simulink model "twip_control_KMLOGIC"  (R2018a)
settings: Solver=ode45  StartTime=0.0  StopTime=10  RelTol=1e-3  EnableMultiTasking=on
values from neighbouring files (symbols this model uses):
  MFM = MFM*length(Centers(i).C)    [Tilt_RuleBase.m]    (also in Yaw_RuleBase.m)
  RulesTILT = [NB NB NB NB NM NS ZR ... (first row only)    [Tilt_RuleBase.m]
  RulesYAW = [NB NB NB NB NM NS ZR ... (first row only)    [Yaw_RuleBase.m]
undefined symbols (not defined in the file or in its folder): CentersTILT, CentersYAW, KMLOGIC
libraries: simulink x2
settings Model: Creator=elew  LastModifiedBy=mattclark
settings DataIOCC: LimitDataPoints=on  SaveFormat=Array
settings OptimizationCC: BlockReduction=off  OptimizeBlockIOStorage=off  BufferReuse=off  GlobalBufferReuse=off  ExpressionFolding=off  LocalBlockOutputs=off  LifeSpan=inf  OptimizeDataStoreBuffers=off  BusAssignmentInplaceUpdate=off
settings DebuggingCC: SFUnexpectedBacktrackingDiag=warning  SFNoUnconditionalDefaultTransitionDiag=warning  SFExecutionAtInitializationDiag=none
settings HardwareCC: ProdBitPerPointer=32  ProdBitPerSizeT=32  ProdBitPerPtrDiffT=32  ProdLargestAtomicFloat=None  ProdIntDivRoundTo=Undefined  ProdEndianess=Unspecified  ProdWordSize=32  ProdHWDeviceType=32-bit Generic
settings ModelReferenceCC: PropagateSignalLabelsOutOfModel=off
settings CodeAppCC: StateflowObjectComments=on
settings GRTTargetCC: TargetLangStandard=C89/C90 (ANSI)  GeneratePreprocessorConditionals=Disable all
settings ConfigComp: CovMetricSettings=dw  CovHtmlReporting=on  CovSaveCumulativeToWorkspaceVar=on  CovSaveSingleToWorkspaceVar=on  CovExternalEMLEnable=off
settings ConfigurationSet: Description=SimMechanics 2G

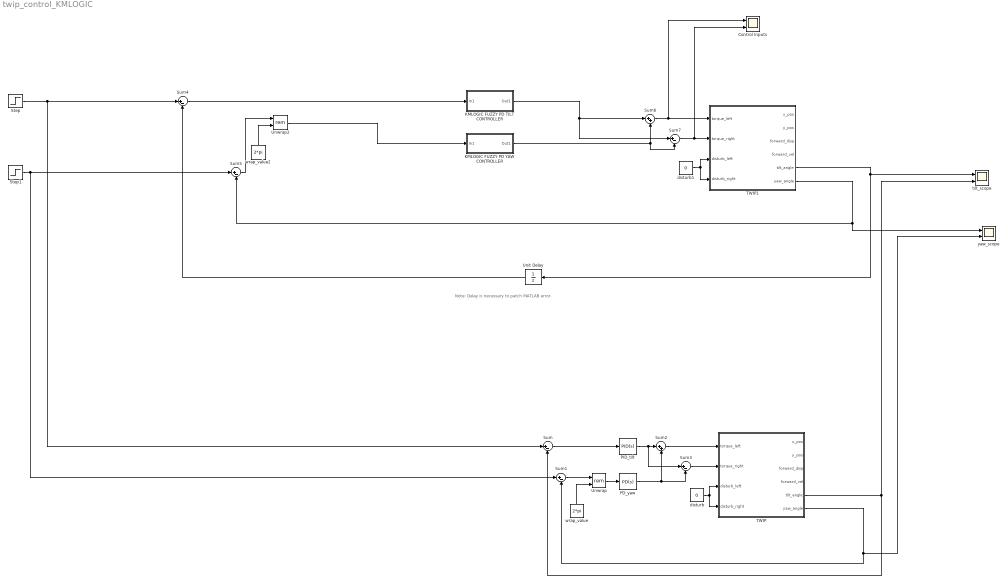
== system twip_control_KMLOGIC ==
  note: Note: Delay is necessary to patch MATLAB error.
  Control Inputs : Scope  NumInputPorts=2
  "KMLOGIC FUZZY PD TILT CONTROLLER " : Subsystem
  KMLOGIC FUZZY PD YAW CONTROLLER : Subsystem
  PD_yaw : simulink/Continuous/PID Controller  Controller=PD  TimeDomain=Continuous-time  SampleTime=-1  IntegratorMethod=Forward Euler  FilterMethod=Forward Euler  Form=Parallel  UseFilter=on  ControllerParametersSource=internal  P=25  I=100  D=1  N=100  InitialConditionSource=internal  InitialConditionForIntegrator=0  InitialConditionForFilter=0  ExternalReset=none  LimitOutput=off  UpperSaturationLimit=inf  LowerSaturationLimit=-inf  LinearizeAsGain=on  AntiWindupMode=none  Kb=1  TrackingMode=off  Kt=1  PParamMin=[]  PParamMax=[]  IParamMin=[]  IParamMax=[]  DParamMin=[]  DParamMax=[]  NParamMin=[]  NParamMax=[]  KbParamMin=[]  KbParamMax=[]  KtParamMin=[]  KtParamMax=[]  POutMin=[]  POutMax=[]  IOutMin=[]  IOutMax=[]  DOutMin=[]  DOutMax=[]  NOutMin=[]  NOutMax=[]  KbOutMin=[]  KbOutMax=[]  KtOutMin=[]  KtOutMax=[]  IntegratorOutMin=[]  IntegratorOutMax=[]  FilterOutMin=[]  FilterOutMax=[]  SumOutMin=[]  SumOutMax=[]  SumI1OutMin=[]  SumI1OutMax=[]  SumI2OutMin=[]  SumI2OutMax=[]  SumI3OutMin=[]  SumI3OutMax=[]  SumDOutMin=[]  SumDOutMax=[]  SaturationOutMin=[]  SaturationOutMax=[]  IntegratorContinuousStateAttributes=''  IntegratorStateMustResolveToSignalObject=off  IntegratorRTWStateStorageClass=Auto  FilterContinuousStateAttributes=''  FilterStateMustResolveToSignalObject=off  FilterRTWStateStorageClass=Auto  DifferentiatorICPrevScaledInput=0  DifferentiatorOutMin=[]  DifferentiatorOutMax=[]  FilterDiffOutCoefMin=[]  FilterDiffOutCoefMax=[]  SumDenOutMin=[]  SumDenOutMax=[]  SumNumOutMin=[]  SumNumOutMax=[]  ReciprocalOutMin=[]  ReciprocalOutMax=[]  DivideOutMin=[]  DivideOutMax=[]  TunerSelectOption=Transfer Function Based (PID Tuner App)
  PID_tilt : simulink/Continuous/PID Controller  Controller=PID  TimeDomain=Continuous-time  SampleTime=-1  IntegratorMethod=Forward Euler  FilterMethod=Forward Euler  Form=Parallel  UseFilter=on  ControllerParametersSource=internal  P=50  I=100  D=2  N=100  InitialConditionSource=internal  InitialConditionForIntegrator=0  InitialConditionForFilter=0  ExternalReset=none  LimitOutput=off  UpperSaturationLimit=inf  LowerSaturationLimit=-inf  LinearizeAsGain=on  AntiWindupMode=none  Kb=1  TrackingMode=off  Kt=1  PParamMin=[]  PParamMax=[]  IParamMin=[]  IParamMax=[]  DParamMin=[]  DParamMax=[]  NParamMin=[]  NParamMax=[]  KbParamMin=[]  KbParamMax=[]  KtParamMin=[]  KtParamMax=[]  POutMin=[]  POutMax=[]  IOutMin=[]  IOutMax=[]  DOutMin=[]  DOutMax=[]  NOutMin=[]  NOutMax=[]  KbOutMin=[]  KbOutMax=[]  KtOutMin=[]  KtOutMax=[]  IntegratorOutMin=[]  IntegratorOutMax=[]  FilterOutMin=[]  FilterOutMax=[]  SumOutMin=[]  SumOutMax=[]  SumI1OutMin=[]  SumI1OutMax=[]  SumI2OutMin=[]  SumI2OutMax=[]  SumI3OutMin=[]  SumI3OutMax=[]  SumDOutMin=[]  SumDOutMax=[]  SaturationOutMin=[]  SaturationOutMax=[]  IntegratorContinuousStateAttributes=''  IntegratorStateMustResolveToSignalObject=off  IntegratorRTWStateStorageClass=Auto  FilterContinuousStateAttributes=''  FilterStateMustResolveToSignalObject=off  FilterRTWStateStorageClass=Auto  DifferentiatorICPrevScaledInput=0  DifferentiatorOutMin=[]  DifferentiatorOutMax=[]  FilterDiffOutCoefMin=[]  FilterDiffOutCoefMax=[]  SumDenOutMin=[]  SumDenOutMax=[]  SumNumOutMin=[]  SumNumOutMax=[]  ReciprocalOutMin=[]  ReciprocalOutMax=[]  DivideOutMin=[]  DivideOutMax=[]  TunerSelectOption=Transfer Function Based (PID Tuner App)
  Step : Step  After=-0.3  SampleTime=0
  Step1 : Step  After=0.1  SampleTime=0
  Sum{,1,3..5,7} (6 alike) : Sum  Inputs=|+-
  Sum2 : Sum  Inputs=|++
  Sum6 : Sum  Inputs=|++
  TWIP : Subsystem
      mask Display:
      | image('twip_mask.png')
      | port_label('input', 1, 'torque_l')
      | port_label('input', 2, 'torque_r')
      | port_label('input', 3, 'disturb_l')
      | port_label('input', 4, 'disturb_r')
      | 
      | 
      | port_label('output', 1, 'x_pos')
      | port_label('output', 2, 'y_pos')
      | port_label('output', 3, 'disp')
      | port_label('output', 4, 'vel')
      | port_label('output', 5, 'tilt')
      | port_label('output', 6, 'yaw')
  TWIP1 : Subsystem
      mask Display:
      | image('twip_mask.png')
      | port_label('input', 1, 'torque_l')
      | port_label('input', 2, 'torque_r')
      | port_label('input', 3, 'disturb_l')
      | port_label('input', 4, 'disturb_r')
      | 
      | 
      | port_label('output', 1, 'x_pos')
      | port_label('output', 2, 'y_pos')
      | port_label('output', 3, 'disp')
      | port_label('output', 4, 'vel')
      | port_label('output', 5, 'tilt')
      | port_label('output', 6, 'yaw')
  Unit Delay : UnitDelay  SampleTime=0.01
  Unwrap : Math  Operator=rem  SaturateOnIntegerOverflow=on
  Unwrap2 : Math  Operator=rem  SaturateOnIntegerOverflow=on
  disturb : Constant  Value=0
  disturb1 : Constant  Value=0
  "tilt_scope " : Scope  NumInputPorts=2
  wrap_value : Constant  Value=2*pi
  wrap_value2 : Constant  Value=2*pi
  yaw_scope : Scope  NumInputPorts=2
  wires:
  TWIP/5(tilt_angle) -> Sum/2, "tilt_scope "/2
  Sum/1 -> PID_tilt/1
  disturb/1 -> TWIP/4(disturb_right), TWIP/3(disturb_left)
  TWIP/6(yaw_angle) -> yaw_scope/2, Sum1/2
  Sum1/1 -> Unwrap/1
  Sum2/1 -> TWIP/1(torque_left)
  Sum3/1 -> TWIP/2(torque_right)
  Unwrap/1 -> PD_yaw/1
  wrap_value/1 -> Unwrap/2
  disturb1/1 -> TWIP1/4(disturb_right), TWIP1/3(disturb_left)
  Sum7/1 -> Control Inputs/2, TWIP1/2(torque_right)
  TWIP1/5(tilt_angle) -> Unit Delay/1, "tilt_scope "/1
  PID_tilt/1 -> Sum3/1, Sum2/1
  Step/1 -> Sum/1, Sum4/1
  Step1/1 -> Sum5/1, Sum1/1
  Sum5/1 -> Unwrap2/1
  Unwrap2/1 -> KMLOGIC FUZZY PD YAW CONTROLLER/1(In1)
  wrap_value2/1 -> Unwrap2/2
  PD_yaw/1 -> Sum3/2, Sum2/2
  Sum6/1 -> Control Inputs/1, TWIP1/1(torque_left)
  KMLOGIC FUZZY PD YAW CONTROLLER/1(Out1) -> Sum7/2, Sum6/2
  TWIP1/6(yaw_angle) -> Sum5/2, yaw_scope/1
  Unit Delay/1 -> Sum4/2
  "KMLOGIC FUZZY PD TILT CONTROLLER "/1(Out1) -> Sum7/1, Sum6/1
  Sum4/1 -> "KMLOGIC FUZZY PD TILT CONTROLLER "/1(In1)

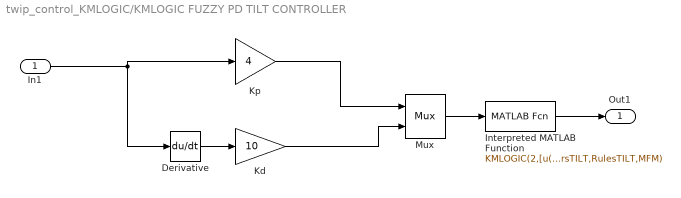
== system twip_control_KMLOGIC/KMLOGIC FUZZY PD TILT CONTROLLER  ==
  In1 : Inport
  Derivative : Derivative
  Interpreted MATLAB Function : MATLABFcn  MATLABFcn=KMLOGIC(2,[u(1), u(2)],CentersTILT,RulesTILT,MFM)  OutputDimensions=1
  "Kd " : Gain  Gain=10
  Kp : Gain  Gain=4
  Mux : Mux  Inputs=2
      settings: DisplayOption=signals
  Out1 : Outport
  wires:
  Derivative/1 -> "Kd "/1
  Kp/1 -> Mux/1
  In1/1 -> Kp/1, Derivative/1
  Interpreted MATLAB Function/1 -> Out1/1
  Mux/1 -> Interpreted MATLAB Function/1
  "Kd "/1 -> Mux/2

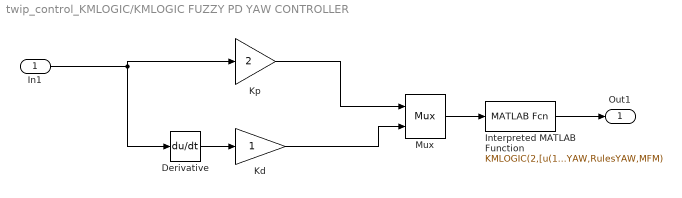
== system twip_control_KMLOGIC/KMLOGIC FUZZY PD YAW CONTROLLER ==
  In1 : Inport
  Derivative : Derivative
  Interpreted MATLAB Function : MATLABFcn  MATLABFcn=KMLOGIC(2,[u(1), u(2)],CentersYAW,RulesYAW,MFM)  OutputDimensions=1
  "Kd " : Gain
  Kp : Gain  Gain=2
  Mux : Mux  Inputs=2
      settings: DisplayOption=signals
  Out1 : Outport
  wires:
  Derivative/1 -> "Kd "/1
  Kp/1 -> Mux/1
  In1/1 -> Kp/1, Derivative/1
  Interpreted MATLAB Function/1 -> Out1/1
  Mux/1 -> Interpreted MATLAB Function/1
  "Kd "/1 -> Mux/2

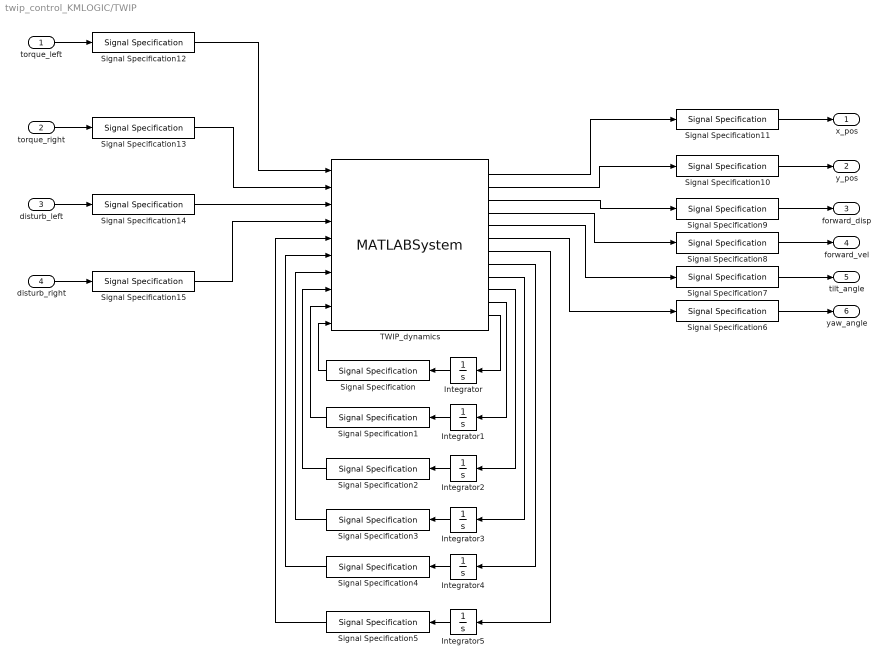
== system twip_control_KMLOGIC/TWIP ==
  torque_left : Inport
  torque_right : Inport  Port=2
  disturb_left : Inport  Port=3
  disturb_right : Inport  Port=4
  Integrator{,1..4} (5 alike) : Integrator
  Integrator5 : Integrator  InitialCondition=0.3
  Signal Specification{,1..15} (16 alike) : SignalSpecification  Dimensions=[1]
  TWIP_dynamics : MATLABSystem  System=twip_sys  M=[0.5]  Mw=[0.8]  mm=[0.5]  Iw=[0.02]  Ip=[0.06]  Imm=[0.08]  r=[0.2]  l=[0.15]  d=[0.6]  SimulateUsing=Interpreted execution
      mask Type: twip_sys
      mask Display:
      | disp('twip_sys');
      | port_label('input',1,'tl');
      | port_label('input',2,'tr');
      | port_label('input',3,'dl');
      | port_label('input',4,'dr');
      | port_label('input',5,'y1');
      | port_label('input',6,'y2');
      | port_label('input',7,'y3');
      | port_label('input',8,'y4');
      | port_label('input',9,'y5');
      | port_label('input',10,'y6');
      | port_label('output',1,'x');
      | port_label('output',2,'y');
      | port_label('output',3,'xp');
      | port_label('output',4,'v');
      | port_label('output',5,'alpha');
      | port_label('output',6,'theta');
      | port_label('output',7,'yd1');
      | port_label('output',8,'yd2');
      | port_label('output',9,'yd3');
      | port_label('output',10,'yd4');
      | port_label('output',11,'yd5');
      | port_label('output',12,'yd6');
  x_pos : Outport
  y_pos : Outport  Port=2
  forward_disp : Outport  Port=3
  forward_vel : Outport  Port=4
  tilt_angle : Outport  Port=5
  yaw_angle : Outport  Port=6
  wires:
  torque_right/1 -> Signal Specification13/1
  torque_left/1 -> Signal Specification12/1
  disturb_right/1 -> Signal Specification15/1
  disturb_left/1 -> Signal Specification14/1
  TWIP_dynamics/1 -> Signal Specification11/1
  TWIP_dynamics/2 -> Signal Specification10/1
  TWIP_dynamics/3 -> Signal Specification9/1
  TWIP_dynamics/4 -> Signal Specification8/1
  TWIP_dynamics/5 -> Signal Specification7/1
  TWIP_dynamics/6 -> Signal Specification6/1
  TWIP_dynamics/12 -> Integrator/1
  Integrator/1 -> Signal Specification/1
  Integrator1/1 -> Signal Specification1/1
  Integrator2/1 -> Signal Specification2/1
  Integrator3/1 -> Signal Specification3/1
  Integrator4/1 -> Signal Specification4/1
  Integrator5/1 -> Signal Specification5/1
  TWIP_dynamics/11 -> Integrator1/1
  TWIP_dynamics/10 -> Integrator2/1
  TWIP_dynamics/9 -> Integrator3/1
  TWIP_dynamics/8 -> Integrator4/1
  TWIP_dynamics/7 -> Integrator5/1
  Signal Specification/1 -> TWIP_dynamics/10
  Signal Specification1/1 -> TWIP_dynamics/9
  Signal Specification2/1 -> TWIP_dynamics/8
  Signal Specification3/1 -> TWIP_dynamics/7
  Signal Specification4/1 -> TWIP_dynamics/6
  Signal Specification5/1 -> TWIP_dynamics/5
  Signal Specification6/1 -> yaw_angle/1
  Signal Specification7/1 -> tilt_angle/1
  Signal Specification8/1 -> forward_vel/1
  Signal Specification9/1 -> forward_disp/1
  Signal Specification10/1 -> y_pos/1
  Signal Specification11/1 -> x_pos/1
  Signal Specification12/1 -> TWIP_dynamics/1
  Signal Specification13/1 -> TWIP_dynamics/2
  Signal Specification14/1 -> TWIP_dynamics/3
  Signal Specification15/1 -> TWIP_dynamics/4

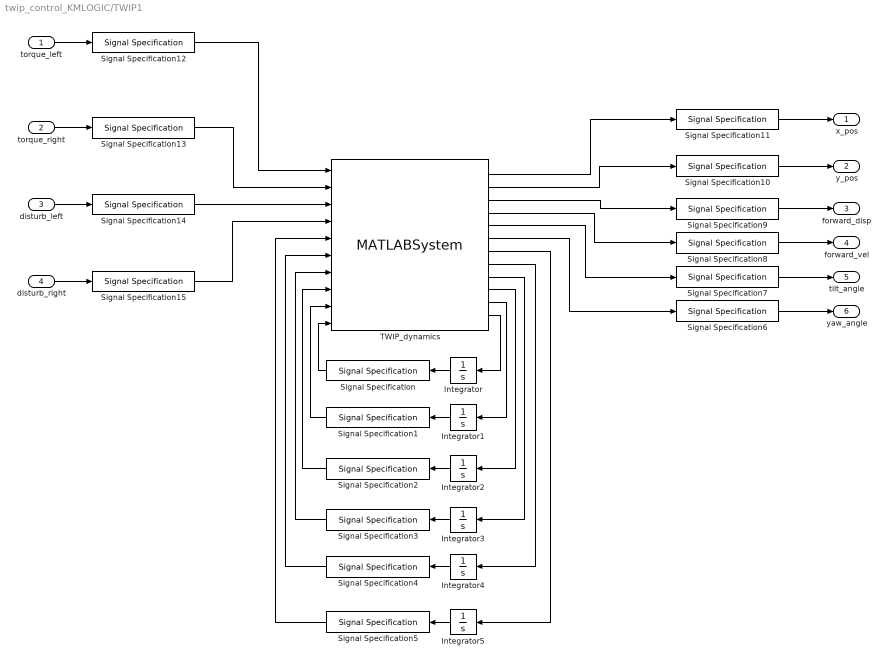
== system twip_control_KMLOGIC/TWIP1 ==
  torque_left : Inport
  torque_right : Inport  Port=2
  disturb_left : Inport  Port=3
  disturb_right : Inport  Port=4
  Integrator{,1..4} (5 alike) : Integrator
  Integrator5 : Integrator  InitialCondition=0.3
  Signal Specification{,1..15} (16 alike) : SignalSpecification  Dimensions=[1]
  TWIP_dynamics : MATLABSystem  System=twip_sys  M=[0.5]  Mw=[0.8]  mm=[0.5]  Iw=[0.02]  Ip=[0.06]  Imm=[0.08]  r=[0.2]  l=[0.15]  d=[0.6]  SimulateUsing=Interpreted execution
      mask Type: twip_sys
      mask Display:
      | disp('twip_sys');
      | port_label('input',1,'tl');
      | port_label('input',2,'tr');
      | port_label('input',3,'dl');
      | port_label('input',4,'dr');
      | port_label('input',5,'y1');
      | port_label('input',6,'y2');
      | port_label('input',7,'y3');
      | port_label('input',8,'y4');
      | port_label('input',9,'y5');
      | port_label('input',10,'y6');
      | port_label('output',1,'x');
      | port_label('output',2,'y');
      | port_label('output',3,'xp');
      | port_label('output',4,'v');
      | port_label('output',5,'alpha');
      | port_label('output',6,'theta');
      | port_label('output',7,'yd1');
      | port_label('output',8,'yd2');
      | port_label('output',9,'yd3');
      | port_label('output',10,'yd4');
      | port_label('output',11,'yd5');
      | port_label('output',12,'yd6');
  x_pos : Outport
  y_pos : Outport  Port=2
  forward_disp : Outport  Port=3
  forward_vel : Outport  Port=4
  tilt_angle : Outport  Port=5
  yaw_angle : Outport  Port=6
  wires:
  torque_right/1 -> Signal Specification13/1
  torque_left/1 -> Signal Specification12/1
  disturb_right/1 -> Signal Specification15/1
  disturb_left/1 -> Signal Specification14/1
  TWIP_dynamics/1 -> Signal Specification11/1
  TWIP_dynamics/2 -> Signal Specification10/1
  TWIP_dynamics/3 -> Signal Specification9/1
  TWIP_dynamics/4 -> Signal Specification8/1
  TWIP_dynamics/5 -> Signal Specification7/1
  TWIP_dynamics/6 -> Signal Specification6/1
  TWIP_dynamics/12 -> Integrator/1
  Integrator/1 -> Signal Specification/1
  Integrator1/1 -> Signal Specification1/1
  Integrator2/1 -> Signal Specification2/1
  Integrator3/1 -> Signal Specification3/1
  Integrator4/1 -> Signal Specification4/1
  Integrator5/1 -> Signal Specification5/1
  TWIP_dynamics/11 -> Integrator1/1
  TWIP_dynamics/10 -> Integrator2/1
  TWIP_dynamics/9 -> Integrator3/1
  TWIP_dynamics/8 -> Integrator4/1
  TWIP_dynamics/7 -> Integrator5/1
  Signal Specification/1 -> TWIP_dynamics/10
  Signal Specification1/1 -> TWIP_dynamics/9
  Signal Specification2/1 -> TWIP_dynamics/8
  Signal Specification3/1 -> TWIP_dynamics/7
  Signal Specification4/1 -> TWIP_dynamics/6
  Signal Specification5/1 -> TWIP_dynamics/5
  Signal Specification6/1 -> yaw_angle/1
  Signal Specification7/1 -> tilt_angle/1
  Signal Specification8/1 -> forward_vel/1
  Signal Specification9/1 -> forward_disp/1
  Signal Specification10/1 -> y_pos/1
  Signal Specification11/1 -> x_pos/1
  Signal Specification12/1 -> TWIP_dynamics/1
  Signal Specification13/1 -> TWIP_dynamics/2
  Signal Specification14/1 -> TWIP_dynamics/3
  Signal Specification15/1 -> TWIP_dynamics/4
